simulink model "mod2_2bit_noDEM"  (Simulink 8.1)
settings: Solver=FixedStepDiscrete  StartTime=0.0  StopTime=100e-3  RelTol=1e-3
undefined symbols (not defined in the file): DACctrl, Fs, modctrl, sinamp, sinfreq
libraries: simulink x3, dspsigops x3, dspsrcs4 x2
settings Model: Creator=amyles  LastModifiedBy=amyles
settings DataIOCC: MaxDataPoints=50000
settings DebuggingCC: StrictBusMsg=Warning
settings SFSimCC: SimParseCustomCode=off

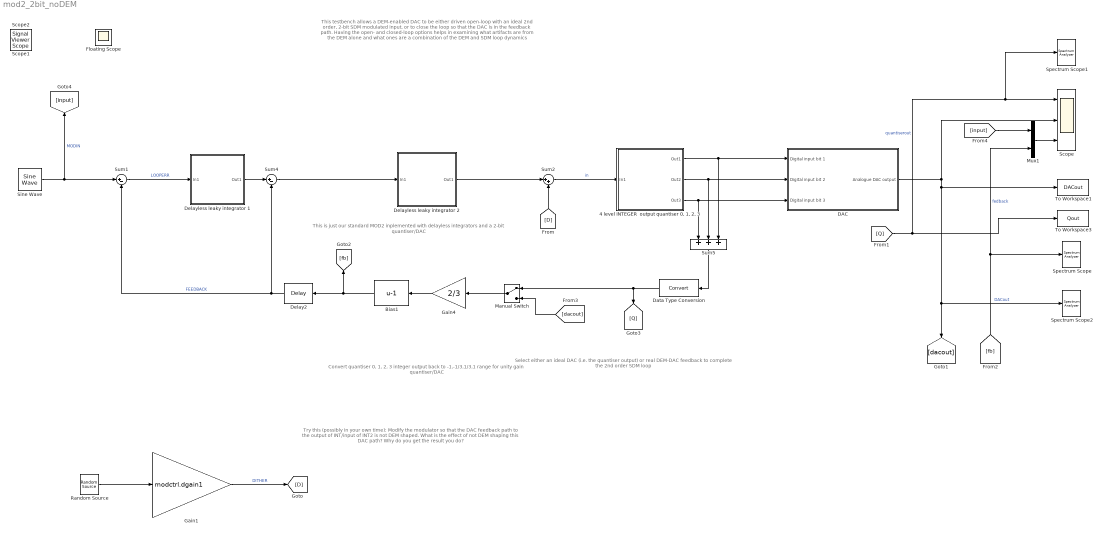
== system mod2_2bit_noDEM ==
  note: Convert quantiser 0, 1, 2, 3 integer
      | output back  to -1,-1/3,1/3,1 range for
      | unity gain quantiser/DAC
  note: Select either an ideal DAC
      | (i.e. the quantiser output) or real
      | DEM-DAC feedback to complete
      | the 2nd order SDM loop
  note: This testbench allows a DEM-enabled DAC to be either driven open-loop with an ideal 2nd order, 2-bit SDM modulated input,
      | or to close the loop so that the DAC is in the feedback path. Having the open- and closed-loop options helps in
      | examining what artifacts are from the DEM alone and what ones are a combination of the DEM and SDM loop dynamics
  note: This is just our standard MOD2 inplemented with delayless integrators and a 2-bit quantiser/DAC
  note: Try this (possibly in your own time):
      | Modify the modulator so that the DAC feedback path to the output of INT/input of INT2 is not DEM shaped.
      | What is the effect of not DEM shaping this DAC path? Why do you get the result you do?
  "4 level INTEGER  output quantiser 0, 1, 2, 3" : Subsystem
  Bias1 : Bias  Bias=-1
  DAC : Subsystem
  Data Type Conversion : DataTypeConversion
  Delay2 : dspsigops/Delay  InputProcessing=Columns as channels (frame based)  dly_unit=Samples  delay=1  ic_detail=off  dif_ic_for_ch=off  dif_ic_for_dly=off  ic=0  reset_popup=None
  Delayless leaky integrator 1 : Subsystem
  Delayless leaky integrator 2 : Subsystem
  Gain1 : Gain  Gain=modctrl.dgain1
      settings: AttributesFormatString=Dither level adjust
  Gain4 : Gain  Gain=2/3
  Manual Switch : ManualSwitch
  Mux1 : Mux  Inputs=2
  Random Source : dspsrcs4/Random Source  SrcType=Uniform  NormMethod=Ziggurat  CltLength=12  MinVal=-1  MaxVal=1  MeanVal=0  VarVal=1  RepMode=Not repeatable  rawSeed=1  IsInherit=off  SampMode=Discrete  SampTime=1/Fs  SampFrame=1  DataType=Double  OutComplex=Real
      settings: AttributesFormatString=Dither source
  Scope : Scope  NumInputPorts=3
      settings: YMin=-5~-5~-5  YMax=5~5~5
  Sine Wave : dspsrcs4/Sine Wave  Amplitude=sinamp  Frequency=sinfreq  Phase=0  SampleMode=Discrete  OutComplex=Real  CompMethod=Trigonometric fcn  TableSize=Speed  SampleTime=1/Fs  SamplesPerFrame=1  ResetState=Restart at time zero  dataType=double  wordLen=16  udDataType=sfix(16)  fracBitsMode=Best precision  numFracBits=15  OutDataTypeStr=double  LastOutDataTypeStr=double
  Spectrum Scope : SpectrumAnalyzer
      settings: CopyFcn=scopeextensions.ScopeBlock.callback(gcbh, 'onBlockCopy', gcbh);  DeleteFcn=scopeextensions.ScopeBlock.callback(gcbh, 'onBlockDelete');  PreSaveFcn=scopeextensions.ScopeBlock.callback(gcbh, 'onModelSave');  NameChangeFcn=scopeextensions.ScopeBlock.callback(gcbh, 'onBlockRename');  CloseFcn=scopeextensions.ScopeBlock.callback(gcbh, 'onBlockClose');  PreDeleteFcn=scopeextensions.ScopeBlock.callback(gcbh, 'onBlockPreDelete');
  Spectrum Scope1 : SpectrumAnalyzer
      settings: CopyFcn=scopeextensions.ScopeBlock.callback(gcbh, 'onBlockCopy', gcbh);  DeleteFcn=scopeextensions.ScopeBlock.callback(gcbh, 'onBlockDelete');  PreSaveFcn=scopeextensions.ScopeBlock.callback(gcbh, 'onModelSave');  NameChangeFcn=scopeextensions.ScopeBlock.callback(gcbh, 'onBlockRename');  CloseFcn=scopeextensions.ScopeBlock.callback(gcbh, 'onBlockClose');  PreDeleteFcn=scopeextensions.ScopeBlock.callback(gcbh, 'onBlockPreDelete');
  Spectrum Scope2 : SpectrumAnalyzer
      settings: CopyFcn=scopeextensions.ScopeBlock.callback(gcbh, 'onBlockCopy', gcbh);  DeleteFcn=scopeextensions.ScopeBlock.callback(gcbh, 'onBlockDelete');  PreSaveFcn=scopeextensions.ScopeBlock.callback(gcbh, 'onModelSave');  NameChangeFcn=scopeextensions.ScopeBlock.callback(gcbh, 'onBlockRename');  CloseFcn=scopeextensions.ScopeBlock.callback(gcbh, 'onBlockClose');  PreDeleteFcn=scopeextensions.ScopeBlock.callback(gcbh, 'onBlockPreDelete');
  Sum1 : Sum  Inputs=|+-
      settings: AttributesFormatString=Modulator input\nloop servo error (input - fbk)
  Sum2 : Sum  Inputs=|++
  Sum4 : Sum  Inputs=|+-
  Sum5 : Sum  Inputs=+++
  To Workspace1 : ToWorkspace  VariableName=DACout  SampleTime=-1
  To Workspace3 : ToWorkspace  VariableName=Qout  SampleTime=-1
  Floating Scope : Scope
      settings: Floating=on
  Scope1 : SignalViewerScope  IOType=viewer  RefreshTime=0.035000
      settings: YMin=-2  YMax=2
  Scope2 : SignalViewerScope  IOType=viewer  NumInputPorts=3  RefreshTime=0.035000
      settings: YMin=-5~-5~-5  YMax=5~5~5
  wires:
  Sum1/1 -> Delayless leaky integrator 1/1(In1)  "LOOPERR"
  Delay2/1 -> Sum1/2, Sum4/2  "FEEDBACK"
  Sine Wave/1 -> Sum1/1, [input]  "MODIN"
  Sum4/1 -> Delayless leaky integrator 2/1(In1)
  Random Source/1 -> Gain1/1
  Gain1/1 -> [D]  "DITHER"
  [D] -> Sum2/2
  Manual Switch/1 -> Gain4/1
  Bias1/1 -> Delay2/1, [fb]
  Gain4/1 -> Bias1/1
  Sum2/1 -> "4 level INTEGER  output quantiser 0, 1, 2, 3"/1(In1)  "in"
  Delayless leaky integrator 1/1(Out1) -> Sum4/1
  Delayless leaky integrator 2/1(Out1) -> Sum2/1
  Data Type Conversion/1 -> Manual Switch/1, [Q]
  [fb] -> Mux1/2, Spectrum Scope/1  "fedback"
  [dacout] -> Manual Switch/2
  [Q] -> Scope/1, Spectrum Scope1/1, To Workspace3/1  "quantiserout"
  "4 level INTEGER  output quantiser 0, 1, 2, 3"/3(Out3) -> Sum5/1, DAC/3(Digital input bit 3)
  "4 level INTEGER  output quantiser 0, 1, 2, 3"/2(Out2) -> Sum5/2, DAC/2(Digital input bit 2)
  Sum5/1 -> Data Type Conversion/1
  "4 level INTEGER  output quantiser 0, 1, 2, 3"/1(Out1) -> Sum5/3, DAC/1(Digital input bit 1)
  DAC/1(Analogue DAC output) -> Scope/2, To Workspace1/1, [dacout], Spectrum Scope2/1  "DACout"
  [input] -> Mux1/1
  Mux1/1 -> Scope/3

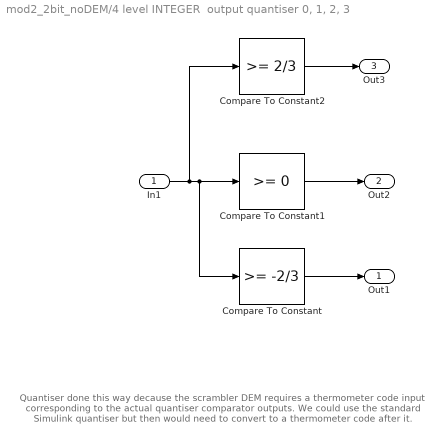
== system mod2_2bit_noDEM/4 level INTEGER  output quantiser 0, 1, 2, 3 ==
  note: Quantiser done this way decause the scrambler DEM
      | requires a thermometer code input corresponding to
      | the actual quantiser comparator outputs. We could use the
      | standard Simulink quantiser but then would need to convert
      | to a thermometer code after it.
  In1 : Inport
  Compare To Constant : simulink/Logic and Bit Operations/Compare To Constant  relop=>=  const=-2/3  OutDataTypeStr=uint8
  Compare To Constant1 : simulink/Logic and Bit Operations/Compare To Constant  relop=>=  const=0  OutDataTypeStr=uint8
  Compare To Constant2 : simulink/Logic and Bit Operations/Compare To Constant  relop=>=  const=2/3  OutDataTypeStr=uint8
  Out1 : Outport
  Out2 : Outport  Port=2
  Out3 : Outport  Port=3
  wires:
  In1/1 -> Compare To Constant/1, Compare To Constant1/1, Compare To Constant2/1
  Compare To Constant/1 -> Out1/1
  Compare To Constant1/1 -> Out2/1
  Compare To Constant2/1 -> Out3/1

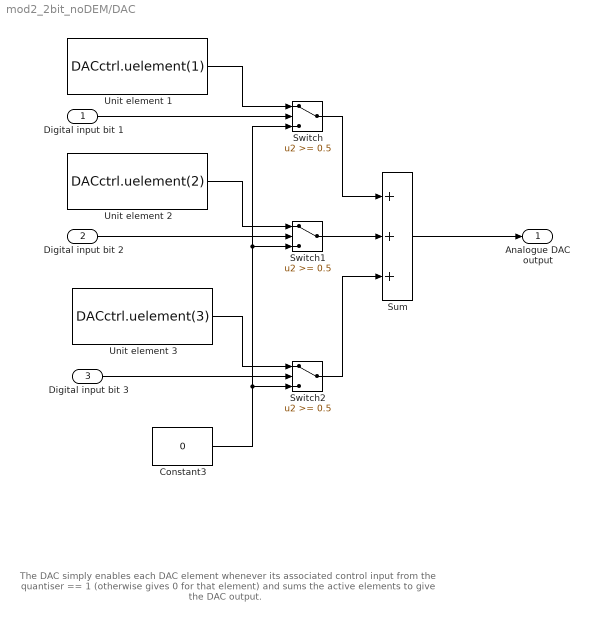
== system mod2_2bit_noDEM/DAC ==
  note: The DAC simply enables each DAC element whenever its associated control
      | input from the quantiser == 1 (otherwise gives 0 for that element)
      | and sums the active elements to give the DAC output.
  Digital input bit 1 : Inport
  Digital input bit 2 : Inport  Port=2
  Digital input bit 3 : Inport  Port=3
  Constant3 : Constant  Value=0  SampleTime=1/Fs
  Sum : Sum  Inputs=+++
  Switch : Switch  Threshold=0.5
  Switch1 : Switch  Threshold=0.5
  Switch2 : Switch  Threshold=0.5
  "Unit element 1 " : Constant  Value=DACctrl.uelement(1)  SampleTime=1/Fs
  Unit element 2 : Constant  Value=DACctrl.uelement(2)  SampleTime=1/Fs
  Unit element 3 : Constant  Value=DACctrl.uelement(3)  SampleTime=1/Fs
  Analogue DAC output : Outport
  wires:
  Switch/1 -> Sum/1
  Switch1/1 -> Sum/2
  Switch2/1 -> Sum/3
  Sum/1 -> Analogue DAC output/1
  Digital input bit 1/1 -> Switch/2
  Digital input bit 2/1 -> Switch1/2
  Digital input bit 3/1 -> Switch2/2
  "Unit element 1 "/1 -> Switch/1
  Constant3/1 -> Switch2/3, Switch1/3, Switch/3
  Unit element 2/1 -> Switch1/1
  Unit element 3/1 -> Switch2/1

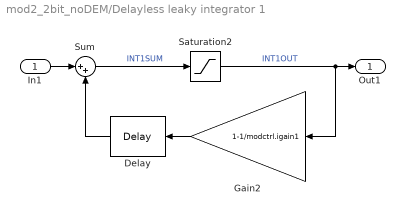
== system mod2_2bit_noDEM/Delayless leaky integrator 1 ==
  In1 : Inport
  Delay : dspsigops/Delay  InputProcessing=Columns as channels (frame based)  dly_unit=Samples  delay=1  ic_detail=off  dif_ic_for_ch=off  dif_ic_for_dly=off  ic=0  reset_popup=None
  Gain2 : Gain  Gain=1-1/modctrl.igain1
      settings: AttributesFormatString=Integrator leakage
  Saturation2 : Saturate  UpperLimit=modctrl.isat1  LowerLimit=-(modctrl.isat1)
  Sum : Sum  Inputs=|++
      settings: AttributesFormatString=Integrator summer
  Out1 : Outport
  wires:
  Delay/1 -> Sum/2
  Sum/1 -> Saturation2/1  "INT1SUM"
  Gain2/1 -> Delay/1
  Saturation2/1 -> Gain2/1, Out1/1  "INT1OUT"
  In1/1 -> Sum/1

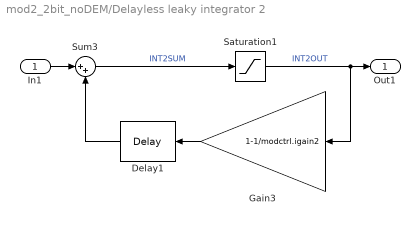
== system mod2_2bit_noDEM/Delayless leaky integrator 2 ==
  In1 : Inport
  Delay1 : dspsigops/Delay  InputProcessing=Columns as channels (frame based)  dly_unit=Samples  delay=1  ic_detail=off  dif_ic_for_ch=off  dif_ic_for_dly=off  ic=0  reset_popup=None
  Gain3 : Gain  Gain=1-1/modctrl.igain2
      settings: AttributesFormatString=Integrator leakage
  Saturation1 : Saturate  UpperLimit=modctrl.isat2  LowerLimit=-(modctrl.isat2)
  Sum3 : Sum  Inputs=|++
      settings: AttributesFormatString=Integrator summer
  Out1 : Outport
  wires:
  Delay1/1 -> Sum3/2
  Sum3/1 -> Saturation1/1  "INT2SUM"
  Gain3/1 -> Delay1/1
  Saturation1/1 -> Gain3/1, Out1/1  "INT2OUT"
  In1/1 -> Sum3/1
